simulink model "leader_qball2"  (Simulink 8.3)
settings: Solver=ode1  StartTime=0.0  StopTime=inf  FixedStep=0.002  RelTol=1e-3
InitFcn:
  | QBall_2_Setup
values from neighbouring files (symbols this model uses):
  g = 9.81    [QBall_2_System_Parameters.m]
  joystick_range_max = 0.8    [QBall_2_Setup.m]
  joystick_range_min = 0.5    [QBall_2_Setup.m]
  KdHEIGHT_DOWN = 0.15    [QBall_2_Controller_Design.m]
  KdHEIGHT_UP = 0.15    [QBall_2_Controller_Design.m]
  KdOUTER_PITCH_DOWN = 0.4    [QBall_2_Controller_Design.m]
  KdOUTER_PITCH_UP = 0.6    [QBall_2_Controller_Design.m]
  KdOUTER_ROLL_DOWN = 0.4    [QBall_2_Controller_Design.m]
  KdOUTER_ROLL_UP = 0.4    [QBall_2_Controller_Design.m]
  KdPITCH_DOWN = 0.1    [QBall_2_Controller_Design.m]
  KdPITCH_UP = 0.1    [QBall_2_Controller_Design.m]
  KdROLL_DOWN = 0.1    [QBall_2_Controller_Design.m]
  KdROLL_UP = 0.1    [QBall_2_Controller_Design.m]
  KdYAW_DOWN = 0.32    [QBall_2_Controller_Design.m]
  KdYAW_UP = 0.32    [QBall_2_Controller_Design.m]
  KiHEIGHT_DOWN = 0.35    [QBall_2_Controller_Design.m]
  KiHEIGHT_UP = 0.35    [QBall_2_Controller_Design.m]
  KiOUTER_PITCH_DOWN = 0.08    [QBall_2_Controller_Design.m]
  KiOUTER_PITCH_UP = 0.08    [QBall_2_Controller_Design.m]
  KiOUTER_ROLL_DOWN = 0.08    [QBall_2_Controller_Design.m]
  KiOUTER_ROLL_UP = 0.08    [QBall_2_Controller_Design.m]
  KiPITCH_DOWN = 0.08    [QBall_2_Controller_Design.m]
  KiPITCH_UP = 0.08    [QBall_2_Controller_Design.m]
  KiROLL_DOWN = 0.08    [QBall_2_Controller_Design.m]
  KiROLL_UP = 0.08    [QBall_2_Controller_Design.m]
  KiYAW_DOWN = 0.0    (= 0)    [QBall_2_Controller_Design.m]
  KiYAW_UP = 0.0    (= 0)    [QBall_2_Controller_Design.m]
  KpHEIGHT_DOWN = 0.5    [QBall_2_Controller_Design.m]
  KpHEIGHT_UP = 0.5    [QBall_2_Controller_Design.m]
  KpOUTER_PITCH_DOWN = 0.3    [QBall_2_Controller_Design.m]
  KpOUTER_PITCH_UP = 0.3    [QBall_2_Controller_Design.m]
  KpOUTER_ROLL_DOWN = 0.3    [QBall_2_Controller_Design.m]
  KpOUTER_ROLL_UP = 0.3    [QBall_2_Controller_Design.m]
  KpPITCH_DOWN = 0.5    [QBall_2_Controller_Design.m]
  KpPITCH_UP = 0.5    [QBall_2_Controller_Design.m]
  KpROLL_DOWN = 0.5    [QBall_2_Controller_Design.m]
  KpROLL_UP = 0.5    [QBall_2_Controller_Design.m]
  KpYAW_DOWN = 0.45    [QBall_2_Controller_Design.m]
  KpYAW_UP = 0.45    [QBall_2_Controller_Design.m]
  LIMIT_CMD_PITCH = 5*pi/180    (= 0.0872664625997)    [QBall_2_Controller_Design.m]
  LIMIT_CMD_ROLL = 5*pi/180    (= 0.0872664625997)    [QBall_2_Controller_Design.m]
  LIMIT_MAX_HEIGHT = 2    [QBall_2_Controller_Design.m]
  LIMIT_MAX_X = 1    [QBall_2_Controller_Design.m]
  LIMIT_MAX_Z = 1    [QBall_2_Controller_Design.m]
  LIMIT_MIN_HEIGHT = 0.3    [QBall_2_Controller_Design.m]
  LIMIT_MIN_X = -1    [QBall_2_Controller_Design.m]
  LIMIT_MIN_Z = -1    [QBall_2_Controller_Design.m]
  LIMIT_RATE_HEIGHT = 0.05    [QBall_2_Controller_Design.m]
  LIMIT_RATE_X = 0.15    [QBall_2_Controller_Design.m]
  LIMIT_RATE_YAW = 15*pi/180    (= 0.261799387799)    [QBall_2_Controller_Design.m]
  LIMIT_RATE_Z = 0.15    [QBall_2_Controller_Design.m]
  LIMIT_uCMD_PITCH = 0.5    [QBall_2_Controller_Design.m]
  LIMIT_uCMD_ROLL = 0.5    [QBall_2_Controller_Design.m]
  LIMIT_uCMD_YAW = 0.5    [QBall_2_Controller_Design.m]
  OFFSET_HEIGHT = 0.3    [QBall_2_System_Parameters.m]
  OMEGA_FILTER = 60    [QBall_2_System_Parameters.m]
  TRIM_THROTTLE = M*g/(4*K)    [QBall_2_Controller_Design.m]
  TRIM_U_PITCH = 0.009    [QBall_2_Controller_Design.m]
  TRIM_U_ROLL = -0.0065    [QBall_2_Controller_Design.m]
undefined symbols (not defined in the file or in its folder): DiscIntNeverNeededParam, qc_get_step_size
libraries: quarc_library x27, simulink x23
(part 1 of 3)
settings Model: Creator=jdaly  LastModifiedBy=user  SimulationMode=external  ExtModeTrigDuration=5000
settings SolverCC: PositivePriorityOrder=on
settings OptimizationCC: ExpressionDepthLimit=2147483647
settings DebuggingCC: FcnCallInpInsideContextMsg=EnableAllAsWarning
settings RTWCC: SystemTargetFile=quarc_linux_duovero.tlc  TemplateMakefile=quarc_linux_duovero_tmf  Description=QUARC Linux DuoVero Target  ProcessScript=quarc_linux_duovero_make_rtw_hook
settings STFCustomTargetCC: TargetLibSuffix=.a  TargetPreCompLibLocation=C:\PROGRA~3\QUARC\lib\2014a\LINUX_~3\release  CodeReplacementLibrary=C89/C90 (ANSI)  ConcurrentExecutionCompliant=on  GeneratePreprocessorConditionals=Disable all  CombineOutputUpdateFcns=on  CPPClassGenCompliant=on  GRTInterface=off  SystemTargetFile=quarc_linux_duovero.tlc
settings GRTTargetCC: TargetLibSuffix=.a  TargetPreCompLibLocation=C:\PROGRA~3\QUARC\lib\2014a\LINUX_~3\release  CodeReplacementLibrary=C89/C90 (ANSI)  ParMdlRefBuildCompliant=off  CompOptLevelCompliant=off  CombineOutputUpdateFcns=on  MatFileLogging=off  GRTInterface=off  ExtMode=on  ExtModeMexFile=quarc_comm  ExtModeMexArgs='-w -d /tmp -uri %u', 'tcpip://192.168.2.26:17001?keep_alive=1'

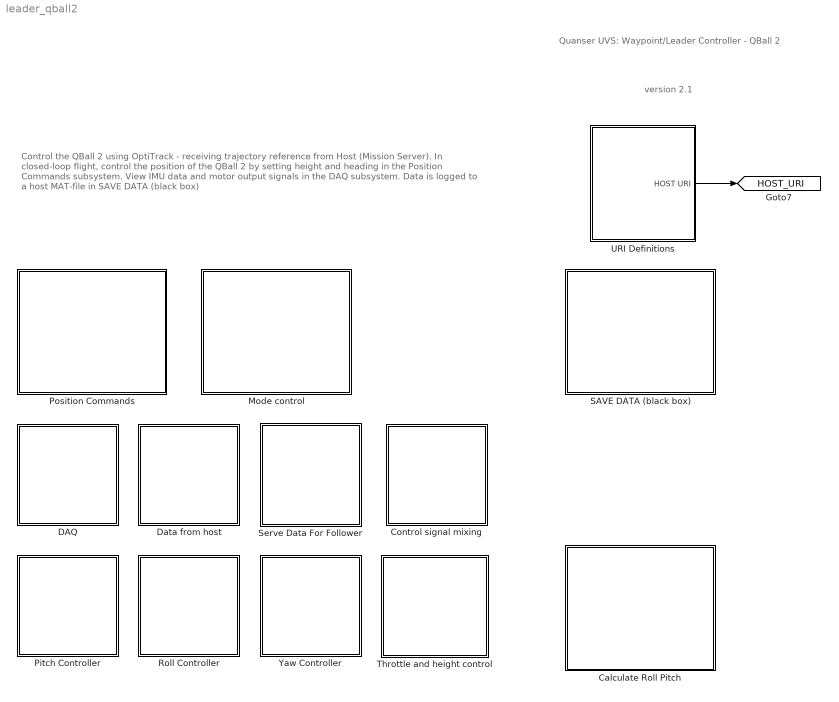
== system leader_qball2 ==
  note: Quanser UVS: Waypoint/Leader Controller - QBall 2
  note: Control the QBall 2 using OptiTrack - receiving trajectory reference
      | from Host (Mission Server).
      |
      | In closed-loop flight, control the position of the QBall 2 by setting height
      | and heading in the Position Commands subsystem.
      |
      | View IMU data and motor output signals in the DAQ subsystem.
      | Data is logged to a host MAT-file in SAVE DATA (black box)
  note: version 2.1
  Calculate Roll Pitch : Subsystem
  Control signal mixing : Subsystem
  DAQ : Subsystem
  Data from host : Subsystem
  Mode control : Subsystem
  Pitch Controller : Subsystem
  Position Commands : Subsystem
  Roll Controller : Subsystem
  SAVE DATA (black box) : Subsystem
  Serve Data For Follower : Subsystem
  Throttle and height control : Subsystem
  URI Definitions : Subsystem
  Yaw Controller : Subsystem
  tag scope: HOST_URI=global
  wires:
  URI Definitions/1(HOST URI) -> [HOST_URI]

== system leader_qball2/Calculate Roll Pitch ==
  note: Note: These calculations are obsolete (as of version 2.1). Roll and Pitch are calculated in the DAQ subsystem.
  Calculate Pitch : Subsystem
  Calculate Roll : Subsystem

== system leader_qball2/Control signal mixing ==
  note: u4 - Right
  note: u3 - Left
  note: u2 - Front
  note: u1 - Back
  Gain2 : Gain  Gain=-1
  Mux : Mux
  Safety - Motor Shutoff if: - Roll/Pitch Data Runaway (> 40 deg) - Initial 3 second of execution for motor initialization : Subsystem
  Sum : Sum  Inputs=+++
  Sum1 : Sum  Inputs=++-
  Sum2 : Sum  Inputs=+++
  Sum3 : Sum  Inputs=++-
  tag scope: motor_outputs=global
  wires:
  Sum1/1 -> Mux/2
  Sum2/1 -> Mux/3
  Sum3/1 -> Mux/4
  Mux/1 -> Safety - Motor Shutoff if: - Roll/Pitch Data Runaway (> 40 deg) - Initial 3 second of execution for motor initialization/1(motors in)
  Sum/1 -> Mux/1
  [u_pitch] -> Sum/3, Sum1/3
  [u_roll] -> Sum2/3, Sum3/3
  [u_yaw] -> Gain2/1, Sum1/2, Sum/2
  Safety - Motor Shutoff if: - Roll/Pitch Data Runaway (> 40 deg) - Initial 3 second of execution for motor initialization/1(motors) -> [motor_outputs]
  Gain2/1 -> Sum2/2, Sum3/2
  [throttle_cmd] -> Sum2/1, Sum3/1, Sum1/1, Sum/1

== system leader_qball2/DAQ ==
  note: Motor outputs: back, front, left, right
  Battery : Scope
      settings: TimeRange=5  YMin=9.9  YMax=13  SaveName=ScopeData14
  Battery (V) : Display
  HIL Initialize : quarc_library/Data Acquisition/Generic/Configuration/HIL Initialize  Priority=-99  object_name=QBall 2  board_type=qball2  board_number=0  board_options=gyro_fs=500;gyro_rate=800;gyro_bw=110;accel_rate=800;accel_fs=8  exclusive=off  active=off  hardware_clocks=[]  clock_modes=[]  initial_clock_frequencies=[]  set_clock_params_at_start=off  set_clock_params_at_switch_in=off  set_clock_frequencies_at_start=off  set_clock_frequencies_at_switch_in=off  analog_input_channels=[0:2]  analog_input_maximums=[5 5 15]  analog_input_minimums=[0 0 0]  set_analog_input_params_at_start=off  set_analog_input_params_at_switch_in=off  analog_output_channels=[]  analog_output_maximums=[]  analog_output_minimums=[]  initial_analog_outputs=[]  final_analog_outputs=[]  watchdog_analog_outputs=[]  set_analog_output_params_at_start=off  set_analog_output_params_at_switch_in=off  set_analog_outputs_at_start=off  set_analog_outputs_at_switch_in=off  set_analog_outputs_at_terminate=off  set_analog_outputs_at_switch_out=off  set_analog_outputs_on_watchdog=off  digital_input_channels=[]  digital_output_channels=[8:9]  digital_output_configuration=[]  initial_digital_outputs=[0]  final_digital_outputs=[1 1]  watchdog_digital_outputs=[0]  set_digital_output_params_at_start=off  set_digital_output_params_at_switch_in=off  set_digital_outputs_at_start=on  set_digital_outputs_at_switch_in=off  set_digital_outputs_at_terminate=on  set_digital_outputs_at_switch_out=off  set_digital_outputs_on_watchdog=on  encoder_channels=[]  quadrature=[]  encoder_filter_frequency=[]  initial_encoder_counts=[]  set_encoder_params_at_start=off  set_encoder_params_at_switch_in=off  set_encoder_counts_at_start=off  set_encoder_counts_at_switch_in=off  pwm_channels=[]  pwm_modes=[0]  pwm_frequency=20e6/1024  pwm_configuration=[0]  pwm_alignment=[0]  pwm_polarity=[1]  pwm_leading_deadband=[0]  pwm_trailing_deadband=[0]  initial_pwm_outputs=[0]  final_pwm_outputs=[0]  watchdog_pwm_outputs=[0]  set_pwm_params_at_start=on  set_pwm_params_at_switch_in=off  set_pwm_outputs_at_start=on  set_pwm_outputs_at_switch_in=off  set_pwm_outputs_at_terminate=on  set_pwm_outputs_at_switch_out=off  set_pwm_outputs_on_watchdog=on  other_output_channels=[11000:11003]  initial_other_outputs=[0]  final_other_outputs=[0]  watchdog_other_outputs=[0]  set_other_outputs_at_start=on  set_other_outputs_at_switch_in=off  set_other_outputs_at_terminate=on  set_other_outputs_at_switch_out=off  set_other_outputs_on_watchdog=on
  HIL Read Write1 : quarc_library/Data Acquisition/Generic/Immediate I//O/HIL Read Write  object_name=QBall 2  analog_output_channels=[]  pwm_output_channels=[]  digital_output_channels=[8, 9]  other_output_channels=[11003 11002 11000:11001]  analog_input_channels=[2]  encoder_input_channels=[]  digital_input_channels=[]  other_input_channels=[3000:3002 4000:4002 0]  sample_time=qc_get_step_size  active=off  vector_output=on  vector_input=on  data_type_mode=Inherit via back propagation  encoder_data_type=double  digital_data_type=boolean
      settings: AttributesFormatString=(%<object_name>)
  HIL Watchdog : quarc_library/Data Acquisition/Generic/Watchdog/HIL Watchdog  object_name=QBall 2  timeout=0.1  sample_time=qc_get_step_size  active=off
      settings: AttributesFormatString=(%<object_name>)
  Initialize sensors : Subsystem
  Low battery check : Subsystem
  Memory : Memory  X0=[0 0 0 0]
  Motor enable : Constant  Value=[1 1]
  PWM : Scope
      settings: TimeRange=5  YMin=0.46  YMax=0.68  SaveName=ScopeData8
  Sample Time : quarc_library/Sources/Time/Sample Time  Priority=-99  sample_time=qc_get_step_size
  Saturation : Saturate  UpperLimit=1  LowerLimit=0
  Select sonar : Selector  InputPortWidth=7  Indices=7
  sonar : Scope
      settings: TimeRange=5  YMin=0.8  YMax=1.4  SaveName=ScopeData34
  spike detection : Subsystem
  watchdog : Scope
      settings: TimeRange=5  YMin=0  YMax=6.5  SaveName=ScopeData32
  tag scope: pwm_output=global, sample_time=global
  wires:
  [motor_outputs] -> Memory/1
  Memory/1 -> Saturation/1
  Saturation/1 -> PWM/1, [pwm_output], HIL Read Write1/2
  Low battery check/1(v) -> Battery (V)/1, Battery/1
  Motor enable/1 -> HIL Read Write1/1
  HIL Read Write1/1 -> Low battery check/1(In1)
  HIL Watchdog/1 -> watchdog/1
  Sample Time/1 -> [sample_time]
  HIL Read Write1/2 -> Select sonar/1, Initialize sensors/1(In1)
  Select sonar/1 -> sonar/1, spike detection/1(In1)

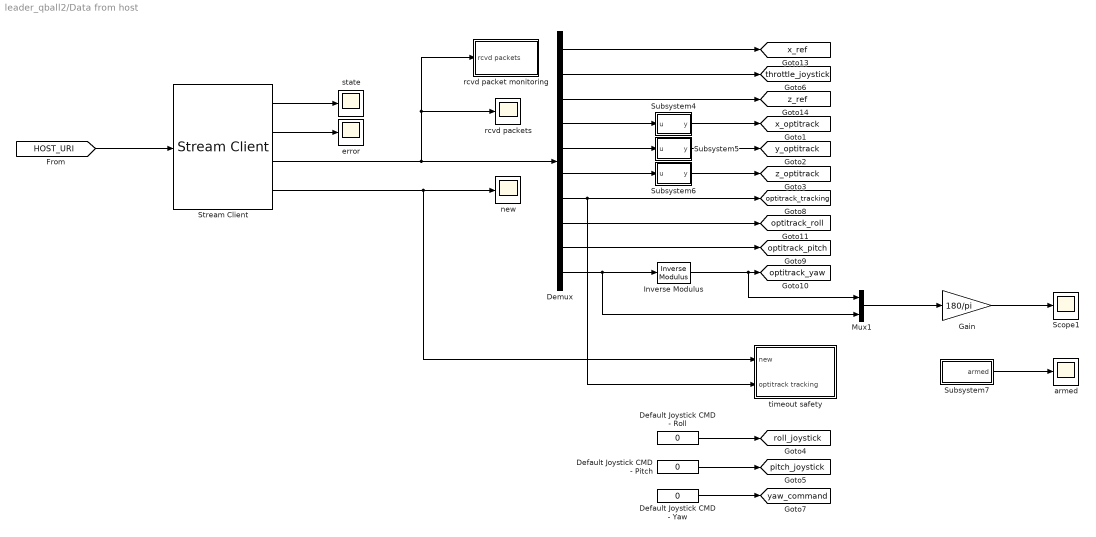
== system leader_qball2/Data from host ==
  Default Joystick CMD - Pitch : Constant  Value=0
  Default Joystick CMD - Roll : Constant  Value=0
  Default Joystick CMD - Yaw : Constant  Value=0
  Demux : Demux  Outputs=10
  Gain : Gain  Gain=180/pi
  Inverse Modulus : quarc_library/Discontinuities/Inverse Modulus  modulus=2*pi  output_derivative=off  output_revolutions=off  max_x=Inf  min_x=-Inf
  Mux1 : Mux  Inputs=2
  Scope1 : Scope
      settings: YMin=-0.48  YMax=-0.405  SaveName=InvModData1
  Stream Client : quarc_library/Communications/Basic/Stream Client  uri_source=External input port  uri=tcpip://192.168.2.15:18005  apply_uri_to_all_configs=on  send_buffer_size=1460  receive_buffer_size=1460  byte_order=little endian (Intel - LSB first)  optimization=Minimum latency  implementation=Use non-blocking I/O  send_options=Do not send data  receive_options=Receive most recent data  send_fifo_size=1000  receive_fifo_size=1000  send_priority=0  receive_priority=0  default_value=zeros(10,1)  send_dimensions=off  receive_dimensions=off  max_dimensions=-1  sample_time=qc_get_step_size  active=off  data_type=Inherited via back propagation  type_expr=BusObject
  Subsystem4 : Subsystem
  Subsystem5 : Subsystem
  Subsystem6 : Subsystem
  Subsystem7 : Subsystem
  armed : Scope
      settings: SaveName=ScopeData7
  error : Scope
      settings: TimeRange=10  YMin=-1  YMax=1  SaveName=ScopeData45
  new : Scope
      settings: SaveName=ScopeData10
  rcvd packet monitoring : Subsystem
  rcvd packets : Scope
      settings: YMin=-1  YMax=1  SaveName=ScopeData5
  state : Scope
      settings: TimeRange=10  YMin=1.9  YMax=2.1  SaveName=ScopeData13
  timeout safety : Subsystem
  tag scope: optitrack_pitch=global, optitrack_roll=global, optitrack_tracking=global, optitrack_yaw=global, pitch_joystick=global, roll_joystick=global, throttle_joystick=global, x_optitrack=global, x_ref=global, y_optitrack=global, yaw_command=global, z_optitrack=global, z_ref=global
  wires:
  Stream Client/1 -> state/1
  Stream Client/2 -> error/1
  Subsystem4/1(y) -> [x_optitrack]
  Subsystem5/1(y) -> [y_optitrack]
  Subsystem6/1(y) -> [z_optitrack]
  Stream Client/3 -> rcvd packets/1, rcvd packet monitoring/1(rcvd packets), Demux/1
  Stream Client/4 -> timeout safety/1(new), new/1
  Subsystem7/1(armed) -> armed/1
  Inverse Modulus/1 -> Mux1/1, [optitrack_yaw]
  Demux/10 -> Mux1/2, Inverse Modulus/1
  Mux1/1 -> Gain/1
  Gain/1 -> Scope1/1
  [HOST_URI] -> Stream Client/1
  Default Joystick CMD - Roll/1 -> [roll_joystick]
  Default Joystick CMD - Pitch/1 -> [pitch_joystick]
  Default Joystick CMD - Yaw/1 -> [yaw_command]
  Demux/9 -> [optitrack_pitch]
  Demux/3 -> [z_ref]
  Demux/2 -> [throttle_joystick]
  Demux/1 -> [x_ref]
  Demux/6 -> Subsystem6/1(u)
  Demux/5 -> Subsystem5/1(u)
  Demux/4 -> Subsystem4/1(u)
  Demux/8 -> [optitrack_roll]
  Demux/7 -> timeout safety/2(optitrack tracking), [optitrack_tracking]

== system leader_qball2/Mode control ==
  note: Note: the height is set to closed-loop mode using the sonar sensor.
      | You can override the height mode and use manual throttle control
      | at your own risk.
  note: Set to 0 for joystick roll and pitch control.
      | Set to 1 for autonomous position control using OptiTrack.
  note: Set to 1 for autonomous heading control using magnetometer.
      | Set to 0 for joystick yaw control.
      | NOTE: first make sure the magnetometer is calibrated and the offset is set in the field
      | HiQ\Calculate Roll Pitch Heading Height\Calculate Heading\camera frame heading offset
  CLOSED-LOOP ON : Constant
  JOYSTICK ON : Constant  Value=0
  Manual Switch2 : ManualSwitch
  Manual Switch4 : ManualSwitch
  tag scope: heading_mode=global, height_mode=global, position_mode=global
  wires:
  CLOSED-LOOP ON/1 -> Manual Switch4/1, Manual Switch2/1, [height_mode]
  JOYSTICK ON/1 -> Manual Switch4/2, Manual Switch2/2
  Manual Switch4/1 -> [heading_mode]
  Manual Switch2/1 -> [position_mode]

== system leader_qball2/Pitch Controller ==
  Gain : Gain  Gain=0.15
  Gain1 : Gain  Gain=180/pi
  Manual Switch : ManualSwitch
  Mux : Mux  Inputs=3
  Mux1 : Mux  Inputs=3
  Pitch : Scope
      settings: YMin=-0.8  YMax=1  SaveName=ScopeData3
  Pitch1 : Scope
      settings: TimeRange=40  YMin=-70  YMax=100  SaveName=ScopeData41
  Subsystem : Subsystem
  pitch controller : Subsystem
  tag scope: pitch_cmd=global
  wires:
  Subsystem/1(pitch command) -> Mux/1, Manual Switch/1
  pitch controller/1(Pitch) -> Mux/2
  Mux/1 -> Pitch/1
  [optitrack_pitch] -> Mux/3
  [pitch_Kalman] -> Mux1/1
  [pitch_comp] -> Mux1/2
  Mux1/1 -> Gain1/1
  Gain1/1 -> Pitch1/1
  [optitrack_pitch] -> Mux1/3
  [pitch_joystick] -> Gain/1
  Manual Switch/1 -> pitch controller/1(cmd), [pitch_cmd]
  Gain/1 -> Manual Switch/2

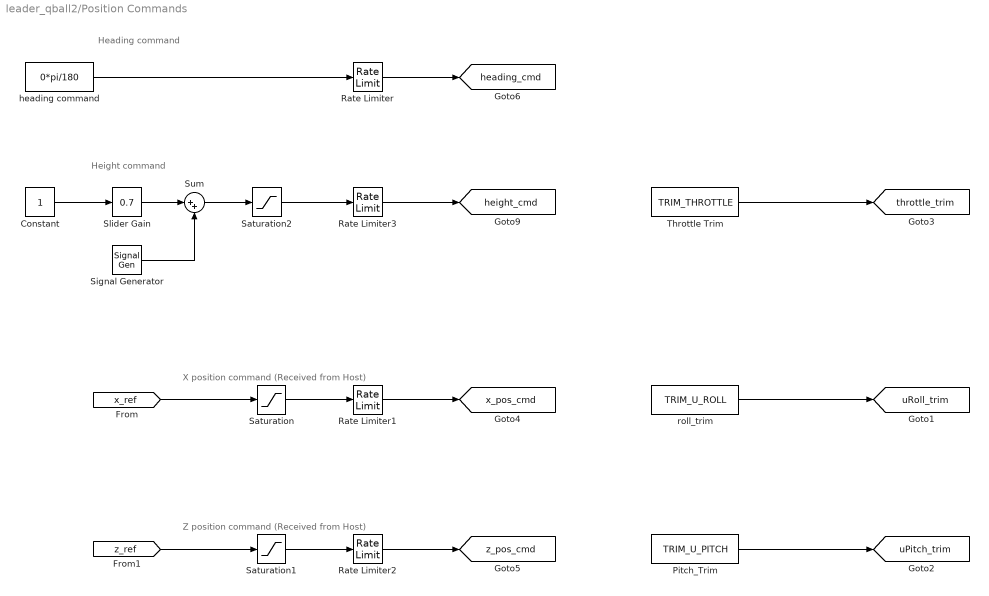
== system leader_qball2/Position Commands ==
  note: Heading command
  note: Height command
  note: X position command (Received from Host)
  note: Z position command (Received from Host)
  Constant : Constant
  Pitch_Trim : Constant  Value=TRIM_U_PITCH
  Rate Limiter : RateLimiter  RisingSlewLimit=LIMIT_RATE_YAW  FallingSlewLimit=-LIMIT_RATE_YAW  SampleTimeMode=inherited
  Rate Limiter1 : RateLimiter  RisingSlewLimit=LIMIT_RATE_X  FallingSlewLimit=-LIMIT_RATE_X  SampleTimeMode=inherited
  Rate Limiter2 : RateLimiter  RisingSlewLimit=LIMIT_RATE_Z  FallingSlewLimit=-LIMIT_RATE_Z  SampleTimeMode=inherited
  Rate Limiter3 : RateLimiter  RisingSlewLimit=LIMIT_RATE_HEIGHT  FallingSlewLimit=-LIMIT_RATE_HEIGHT  SampleTimeMode=inherited
  Saturation : Saturate  UpperLimit=LIMIT_MAX_X  LowerLimit=LIMIT_MIN_X
  Saturation1 : Saturate  UpperLimit=LIMIT_MAX_Z  LowerLimit=LIMIT_MIN_Z
  Saturation2 : Saturate  UpperLimit=LIMIT_MAX_HEIGHT  LowerLimit=LIMIT_MIN_HEIGHT
  Signal Generator : SignalGenerator  WaveForm=square  Amplitude=0  Frequency=0.0125
  Slider Gain : simulink/Math Operations/Slider Gain  low=0  gain=0.7  high=1
  Sum : Sum  Inputs=|++
  Throttle Trim : Constant  Value=TRIM_THROTTLE
  heading command : Constant  Value=0*pi/180
  roll_trim : Constant  Value=TRIM_U_ROLL
  tag scope: heading_cmd=global, height_cmd=global, throttle_trim=global, uPitch_trim=global, uRoll_trim=global, x_pos_cmd=global, z_pos_cmd=global
  wires:
  Saturation/1 -> Rate Limiter1/1
  Saturation1/1 -> Rate Limiter2/1
  Constant/1 -> Slider Gain/1
  heading command/1 -> Rate Limiter/1
  Slider Gain/1 -> Sum/1
  Sum/1 -> Saturation2/1
  Signal Generator/1 -> Sum/2
  Rate Limiter/1 -> [heading_cmd]
  Saturation2/1 -> Rate Limiter3/1
  Rate Limiter1/1 -> [x_pos_cmd]
  Rate Limiter2/1 -> [z_pos_cmd]
  Rate Limiter3/1 -> [height_cmd]
  Throttle Trim/1 -> [throttle_trim]
  roll_trim/1 -> [uRoll_trim]
  Pitch_Trim/1 -> [uPitch_trim]
  [x_ref] -> Saturation/1
  [z_ref] -> Saturation1/1

== system leader_qball2/Roll Controller ==
  Gain : Gain  Gain=0.15
  Gain1 : Gain  Gain=180/pi
  Gain4 : Gain  Gain=180/pi
  Manual Switch : ManualSwitch
  Mux : Mux
  Mux1 : Mux
  Roll : Scope
      settings: TimeRange=40  YMin=0  YMax=47.5  SaveName=ScopeData9
  Roll Controller : Subsystem
  Roll1 : Scope
      settings: TimeRange=40  YMin=-60  YMax=100  SaveName=ScopeData40
  Subsystem : Subsystem
  tag scope: roll_cmd=global
  wires:
  Subsystem/1(roll command) -> Mux/1, Manual Switch/1
  Mux/1 -> Gain4/1
  Roll Controller/1(Roll) -> Mux/2
  [optitrack_roll] -> Mux/3
  [roll_Kalman] -> Mux/4
  Gain4/1 -> Roll/1
  [roll_Kalman] -> Mux1/1
  [roll_comp] -> Mux1/2
  Mux1/1 -> Gain1/1
  Gain1/1 -> Roll1/1
  [optitrack_roll] -> Mux1/3
  [roll_acc] -> Mux1/4
  Manual Switch/1 -> [roll_cmd], Roll Controller/1(cmd)
  [roll_joystick] -> Gain/1
  Gain/1 -> Manual Switch/2

== system leader_qball2/SAVE DATA (black box) ==
  note: Saves the data to a MAT file on the host PC. Note that the model must be connected
      | in external mode and stopped correctly for the MAT file to be saved.
      | Append signals to the end of the mux block to save additional signals.
      | Each time the model is run it saves a new file with the data and time appended
      | to the file name.
      |
      | Signals can be read after stopping the model by first loading the MAT file, then plotting
      | the data signals. NOTE: data points are saved in rows, with the first row always containing
      | the time signal - so add 1 to the index of the signals listed here. E.g.,
      |
      | load qball_flight_data.mat
      | t = qball_data(1,:);
      | roll = qball_data(22,:);
      | plot(t, roll);
  Mux1 : Mux  Inputs=7
  Signals 1-10 : Subsystem
  Signals 11-20 : Subsystem
  Signals 21-30 : Subsystem
  Signals 31-40 : Subsystem
  Signals 41-50 : Subsystem
  Signals 51-60 : Subsystem
  Signals 61-70 : Subsystem
  To Host File : quarc_library/Sinks/To Host/To Host File  file_name=qball_flight_data_%{date}_%{time}.mat  variable_name=qball_data  decimation=1  sample_time=-1  file_format=MAT-file v.4  options=No header or footer  append=off  final_file_name=qball_flight_data_20-Aug-2015_16-55-50.mat
      settings: AttributesFormatString=%<file_name>
  wires:
  Mux1/1 -> To Host File/1
  Signals 41-50/1(Out1) -> Mux1/5
  Signals 31-40/1(Out1) -> Mux1/4
  Signals 21-30/1(Out1) -> Mux1/3
  Signals 11-20/1(Out1) -> Mux1/2
  Signals 1-10/1(Out1) -> Mux1/1
  Signals 51-60/1(Out1) -> Mux1/6
  Signals 61-70/1(Out1) -> Mux1/7

== system leader_qball2/Serve Data For Follower ==
  Display1 : Display
      settings: Decimation=100
  Display2 : Display
      settings: Decimation=100
  Display3 : Display
      settings: Decimation=100
  Dummy Heading Reference (rad) : Constant  Value=0
  Enable : Constant
  Mux : Mux  Inputs=3
  Stream Server : quarc_library/Communications/Basic/Stream Server  uri_source=Specify via dialog (do not evaluate)  uri=tcpip://localhost:18007  apply_uri_to_all_configs=on  send_buffer_size=1460  receive_buffer_size=1460  byte_order=little endian (Intel - LSB first)  optimization=Minimum latency  implementation=Use non-blocking I/O  send_options=Send most recent data  receive_options=Do not receive data  send_fifo_size=1000  receive_fifo_size=1000  send_priority=0  receive_priority=0  default_value=[0]  send_dimensions=off  receive_dimensions=off  max_dimensions=-1  sample_time=qc_get_step_size  active=off  data_type=Inherited via back propagation  type_expr=BusObject
      settings: AttributesFormatString="\"tcpip://localhost:18007\""
  wires:
  Mux/1 -> Stream Server/1
  Enable/1 -> Stream Server/2
  Stream Server/3 -> Display3/1
  Stream Server/2 -> Display2/1
  Stream Server/1 -> Display1/1
  [z_optitrack] -> Mux/2
  [x_optitrack] -> Mux/1
  Dummy Heading Reference (rad)/1 -> Mux/3

== system leader_qball2/Throttle and height control ==
  Height joystick adjust : Subsystem
  Joystick mode throttle : Subsystem
  "Safety - Active During Emergency Landing: Ramp Throttle CMD down to zero if Sonar Failed " : Subsystem
  Switch : Switch  Threshold=0.5
  height control : Subsystem
  throttle cmd : Scope
      settings: YMin=0  YMax=1.1  SaveName=ScopeData19
  throttle sw : Scope
      settings: YMin=0.05  YMax=0.1  SaveName=ScopeData27
  tag scope: throttle_cmd=global
  wires:
  Height joystick adjust/1(cmd out) -> height control/1(height command)
  Switch/1 -> throttle sw/1, "Safety - Active During Emergency Landing: Ramp Throttle CMD down to zero if Sonar Failed "/1(throttle)
  height control/1(throttle) -> Switch/1
  Joystick mode throttle/1(throttle) -> Switch/3
  [height_mode] -> Switch/2
  "Safety - Active During Emergency Landing: Ramp Throttle CMD down to zero if Sonar Failed "/1(Out1) -> throttle cmd/1, [throttle_cmd]
  [height_cmd] -> Height joystick adjust/1(cmd)

== system leader_qball2/URI Definitions ==
  note: Note: Make sure QBall 2 IP address match the intended active unit in the following places:
      | - Under Simulation->Model Configuration Parameters->Code Generation->Interface->MEX-file arguments
  note: Default URI:
      |
      | HOST Server to LEADER: tcpip://192.168.2.222:18006
      | HOST Server to FOLLOWER: tcpip://192.168.2.222:18005
      | LEADER Server to FOLLOWER: tcpip://192.168.30:18007
      |
      | Leader/Waypoint Control Model URI:
      | tcpip://192.168.2.22:17001?nagle=no,keep_alive=1
  note: Define Communications URI Here
  String Constant1 : quarc_library/Strings/String Constant  string_value=tcpip://192.168.2.10:18006  evaluate_string=off  string_type=text  max_length=80  sample_time=inf  variable_size=off
      settings: AttributesFormatString="\"tcpip://192.168.2.10:18006\""
  HOST URI : Outport
  wires:
  String Constant1/1 -> HOST URI/1

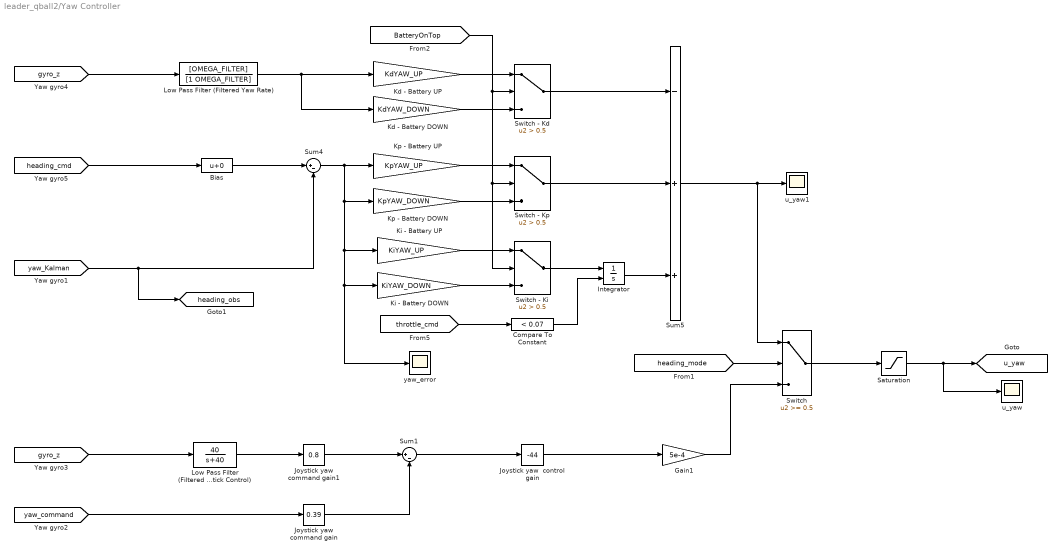
== system leader_qball2/Yaw Controller ==
  Bias : Bias
  Compare To Constant : simulink/Logic and Bit Operations/Compare To Constant  relop=<  const=0.07  OutDataTypeStr=boolean  ZeroCross=off
  Gain1 : Gain  Gain=5e-4
  Integrator : Integrator  ExternalReset=level
  Joystick yaw  control gain : simulink/Math Operations/Slider Gain  low=-100  gain=-44  high=0
  Joystick yaw command gain : simulink/Math Operations/Slider Gain  low=0  gain=0.39  high=0.6
  Joystick yaw command gain1 : simulink/Math Operations/Slider Gain  low=-1  gain=0.8  high=1
  Kd - Battery DOWN : Gain  Gain=KdYAW_DOWN
  Kd - Battery UP : Gain  Gain=KdYAW_UP
  Ki - Battery DOWN : Gain  Gain=KiYAW_DOWN
  Ki - Battery UP : Gain  Gain=KiYAW_UP
  Kp - Battery DOWN : Gain  Gain=KpYAW_DOWN
  Kp - Battery UP : Gain  Gain=KpYAW_UP
  Low Pass Filter (Filtered Yaw Rate) : TransferFcn  Numerator=[OMEGA_FILTER]  Denominator=[1 OMEGA_FILTER]
  Low Pass Filter (Filtered Yaw Rate) (For Joytstick Control) : TransferFcn  Numerator=[40]  Denominator=[1 40]
  Saturation : Saturate  UpperLimit=LIMIT_uCMD_YAW  LowerLimit=-LIMIT_uCMD_YAW
  Sum1 : Sum  Inputs=|+-
  Sum4 : Sum  Inputs=|+-
  Sum5 : Sum  Inputs=-++
  Switch : Switch  Threshold=0.5
  Switch - Kd : Switch  Criteria=u2 > Threshold  Threshold=0.5
  Switch - Ki : Switch  Criteria=u2 > Threshold  Threshold=0.5
  Switch - Kp : Switch  Criteria=u2 > Threshold  Threshold=0.5
  u_yaw : Scope
      settings: YMin=-0.0225  YMax=0.02  SaveName=ScopeData4
  u_yaw1 : Scope
      settings: YMin=2.93e-05  YMax=3.15e-05  SaveName=ScopeData23
  yaw_error : Scope
      settings: YMin=-0.1005  YMax=-0.091  SaveName=ScopeData24
  tag scope: heading_obs=global, u_yaw=global
  wires:
  [yaw_command] -> Joystick yaw command gain/1
  Sum1/1 -> Joystick yaw  control gain/1
  [heading_mode] -> Switch/2
  Switch/1 -> Saturation/1
  Joystick yaw command gain/1 -> Sum1/2
  Joystick yaw  control gain/1 -> Gain1/1
  Gain1/1 -> Switch/3
  Sum4/1 -> Kp - Battery DOWN/1, Ki - Battery UP/1, Ki - Battery DOWN/1, yaw_error/1, Kp - Battery UP/1
  Sum5/1 -> Switch/1, u_yaw1/1
  [yaw_Kalman] -> Sum4/2, [heading_obs]
  Saturation/1 -> [u_yaw], u_yaw/1
  [gyro_z] -> Low Pass Filter (Filtered Yaw Rate) (For Joytstick Control)/1
  Low Pass Filter (Filtered Yaw Rate) (For Joytstick Control)/1 -> Joystick yaw command gain1/1
  Joystick yaw command gain1/1 -> Sum1/1
  [heading_cmd] -> Bias/1
  Compare To Constant/1 -> Integrator/2
  [throttle_cmd] -> Compare To Constant/1
  [gyro_z] -> Low Pass Filter (Filtered Yaw Rate)/1
  Low Pass Filter (Filtered Yaw Rate)/1 -> Kd - Battery UP/1, Kd - Battery DOWN/1
  Integrator/1 -> Sum5/3
  Bias/1 -> Sum4/1
  Kd - Battery UP/1 -> Switch - Kd/1
  Kd - Battery DOWN/1 -> Switch - Kd/3
  [BatteryOnTop] -> Switch - Kp/2, Switch - Ki/2, Switch - Kd/2
  Kp - Battery UP/1 -> Switch - Kp/1
  Kp - Battery DOWN/1 -> Switch - Kp/3
  Switch - Kd/1 -> Sum5/1
  Switch - Kp/1 -> Sum5/2
  Ki - Battery UP/1 -> Switch - Ki/1
  Ki - Battery DOWN/1 -> Switch - Ki/3
  Switch - Ki/1 -> Integrator/1

== system leader_qball2/Calculate Roll Pitch/Calculate Pitch ==
  Fcn : Fcn  Expr=asin(u/9.81)
  HPF : TransferFcn  Numerator=[2 0]  Denominator=[2 1]
  Integrator : Integrator
  LPF : TransferFcn  Numerator=1  Denominator=[2 1]
  Sum2 : Sum
  Terminator : Terminator
  tag scope: pitch=global, pitch_comp=global
  wires:
  [accel_x] -> Fcn/1
  Integrator/1 -> HPF/1
  HPF/1 -> Sum2/2, [pitch_comp]
  LPF/1 -> Sum2/1
  Fcn/1 -> [pitch], LPF/1
  [gyro_y] -> Integrator/1
  Sum2/1 -> Terminator/1

== system leader_qball2/Calculate Roll Pitch/Calculate Roll ==
  Fcn : Fcn  Expr=asin(u/9.81)
  Gain1 : Gain  Gain=-1
  HPF1 : TransferFcn  Numerator=[2 0]  Denominator=[2 1]
  Integrator : Integrator
  LPF1 : TransferFcn  Numerator=1  Denominator=[2 1]
  Manual Switch : ManualSwitch
  Sum3 : Sum
  Switch : Switch  Threshold=0.5
  Terminator : Terminator
  tag scope: roll=global, roll_comp=global
  wires:
  [accel_y] -> Gain1/1
  Gain1/1 -> Fcn/1
  [gyro_x] -> Integrator/1
  Integrator/1 -> HPF1/1
  Fcn/1 -> LPF1/1, [roll]
  LPF1/1 -> Sum3/1
  HPF1/1 -> Sum3/2, Manual Switch/1
  [optitrack_tracking] -> Switch/2
  Sum3/1 -> Switch/3
  [optitrack_roll] -> Switch/1
  Switch/1 -> Terminator/1
  Manual Switch/1 -> [roll_comp]
  [roll_acc] -> Manual Switch/2

== system leader_qball2/Control signal mixing/Safety - Motor Shutoff if: - Roll/Pitch Data Runaway (> 40 deg) - Initial 3 second of execution for motor initialization ==
  note: Check that pitch and roll are always less than 40 degrees.
      | If pitch or roll exceeds 40 degrees it is a runaway condition
      | and the motors should be stopped.
  motors in : Inport
  Abs : Abs
  Abs1 : Abs
  Compare To Constant1 : simulink/Logic and Bit Operations/Compare To Constant  relop=>  const=40*pi/180  OutDataTypeStr=uint8  ZeroCross=off
  Compare To Constant2 : simulink/Logic and Bit Operations/Compare To Constant  relop=>  const=40*pi/180  OutDataTypeStr=uint8  ZeroCross=off
  Enabled Subsystem : Subsystem  TreatAsAtomicUnit=on
  Logical Operator : Logic  Operator=OR  AllPortsSameDT=off  OutDataTypeStr=boolean
  Product1 : Product  Inputs=3  OutDataTypeStr=double  RndMeth=Zero
  Product2 : Product  OutDataTypeStr=double  RndMeth=Zero
  "Roll, Pitch runaway check" : Scope
      settings: SaveName=ScopeData38
  Step Initialize zero throttle for 3 seconds : Step  Time=3  SampleTime=0
  motors_in : Scope
      settings: SaveName=ScopeData50
  motors_out : Scope
      settings: SaveName=ScopeData51
  throttle enable : Subsystem
  motors : Outport
  wires:
  motors in/1 -> motors_in/1, Product1/2
  throttle enable/1(en) -> Product1/1
  [roll_comp] -> Abs1/1
  [pitch_comp] -> Abs/1
  Compare To Constant1/1 -> Logical Operator/1
  Compare To Constant2/1 -> Logical Operator/2
  Logical Operator/1 -> Enabled Subsystem/Enable
  Enabled Subsystem/1(Out1) -> "Roll, Pitch runaway check"/1, Product1/3
  Product1/1 -> Product2/2
  Abs/1 -> Compare To Constant1/1
  Abs1/1 -> Compare To Constant2/1
  Step Initialize zero throttle for 3 seconds/1 -> Product2/1
  Product2/1 -> motors_out/1, motors/1

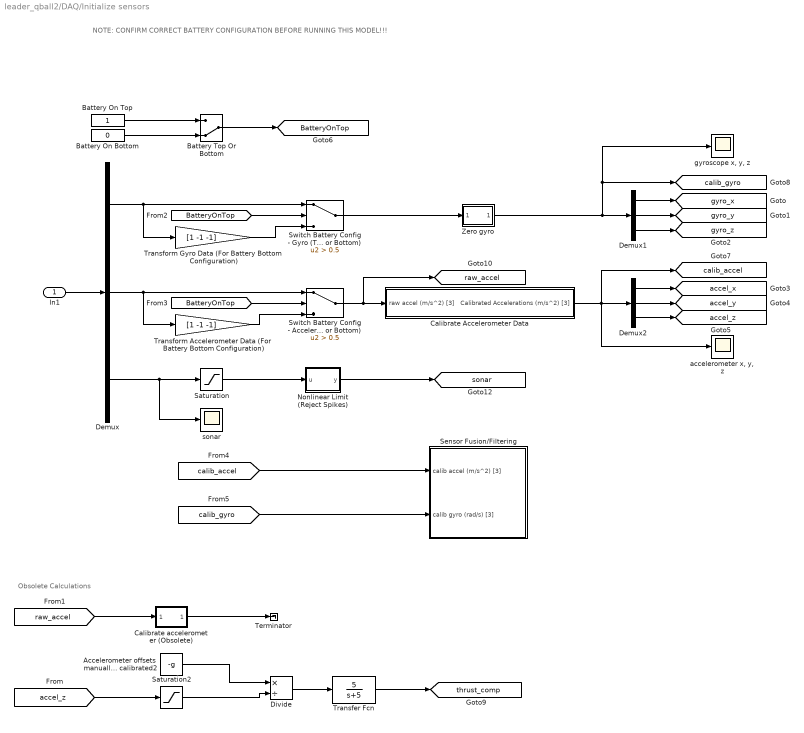
== system leader_qball2/DAQ/Initialize sensors ==
  note: Obsolete Calculations
  note: NOTE: CONFIRM CORRECT BATTERY
      | CONFIGURATION BEFORE RUNNING
      | THIS MODEL!!!
  In1 : Inport
  Accelerometer offsets manually calibrated2 : Constant  Value=-g
  Battery On Bottom : Constant  Value=0
  Battery On Top : Constant
  Battery Top Or Bottom : ManualSwitch  CurrentSetting=0
  Calibrate Accelerometer Data : Subsystem
  Calibrate accelerometer (Obsolete) : Subsystem
  Demux : Demux  Outputs=[3 3 1]
  Demux1 : Demux  Outputs=3
  Demux2 : Demux  Outputs=3
  Divide : Product  Inputs=*/
  Nonlinear Limit (Reject Spikes) : Subsystem
  Saturation : Saturate  UpperLimit=3  LowerLimit=0
  Saturation2 : Saturate  UpperLimit=-9.0  LowerLimit=-9.8
  Sensor Fusion/Filtering : Subsystem
  Switch Battery Config - Acceleromter (Top or Bottom) : Switch  Criteria=u2 > Threshold  Threshold=0.5
  Switch Battery Config - Gyro (Top or Bottom) : Switch  Criteria=u2 > Threshold  Threshold=0.5
  Terminator : Terminator
  Transfer Fcn : TransferFcn  Numerator=[5]  Denominator=[1 5]
  Transform Accelerometer Data (For Battery Bottom Configuration) : Gain  Gain=[1 -1 -1]
  Transform Gyro Data (For Battery Bottom Configuration) : Gain  Gain=[1 -1 -1]
  Zero gyro : Subsystem
  "accelerometer x, y, z" : Scope
      settings: TimeRange=5  YMin=-10  YMax=3  SaveName=ScopeData31
  "gyroscope x, y, z" : Scope
      settings: TimeRange=5  YMin=-0.125  YMax=0.425  SaveName=ScopeData30
  sonar : Scope
      settings: YMin=0.1  YMax=1.9  SaveName=ScopeData15
  tag scope: BatteryOnTop=global, accel_x=global, accel_y=global, accel_z=global, calib_accel=global, calib_gyro=global, gyro_x=global, gyro_y=global, gyro_z=global, raw_accel=global, sonar=global, thrust_comp=global
  wires:
  Demux1/1 -> [gyro_x]
  Demux1/2 -> [gyro_y]
  Demux1/3 -> [gyro_z]
  Demux2/1 -> [accel_x]
  Demux2/2 -> [accel_y]
  Demux2/3 -> [accel_z]
  Accelerometer offsets manually calibrated2/1 -> Divide/1
  Divide/1 -> Transfer Fcn/1
  Transfer Fcn/1 -> [thrust_comp]
  In1/1 -> Demux/1
  Saturation/1 -> Nonlinear Limit (Reject Spikes)/1(u)
  Nonlinear Limit (Reject Spikes)/1(y) -> [sonar]
  Saturation2/1 -> Divide/2
  [accel_z] -> Saturation2/1
  [raw_accel] -> Calibrate accelerometer (Obsolete)/1(In1)
  Calibrate accelerometer (Obsolete)/1(Out1) -> Terminator/1
  Demux/3 -> sonar/1, Saturation/1
  [BatteryOnTop] -> Switch Battery Config - Gyro (Top or Bottom)/2
  Transform Gyro Data (For Battery Bottom Configuration)/1 -> Switch Battery Config - Gyro (Top or Bottom)/3
  Demux/2 -> Switch Battery Config - Acceleromter (Top or Bottom)/1, Transform Accelerometer Data (For Battery Bottom Configuration)/1
  [BatteryOnTop] -> Switch Battery Config - Acceleromter (Top or Bottom)/2
  Transform Accelerometer Data (For Battery Bottom Configuration)/1 -> Switch Battery Config - Acceleromter (Top or Bottom)/3
  Switch Battery Config - Gyro (Top or Bottom)/1 -> Zero gyro/1(In1)
  [calib_gyro] -> Sensor Fusion/Filtering/2(calib gyro (rad/s) [3])
  [calib_accel] -> Sensor Fusion/Filtering/1(calib accel (m/s^2) [3])
  Switch Battery Config - Acceleromter (Top or Bottom)/1 -> [raw_accel], Calibrate Accelerometer Data/1(raw accel (m/s^2) [3])
  Demux/1 -> Transform Gyro Data (For Battery Bottom Configuration)/1, Switch Battery Config - Gyro (Top or Bottom)/1
  Zero gyro/1(Out1) -> Demux1/1, "gyroscope x, y, z"/1, [calib_gyro]
  Calibrate Accelerometer Data/1(Calibrated Accelerations (m/s^2) [3]) -> "accelerometer x, y, z"/1, Demux2/1, [calib_accel]
  Battery On Bottom/1 -> Battery Top Or Bottom/2
  Battery On Top/1 -> Battery Top Or Bottom/1
  Battery Top Or Bottom/1 -> [BatteryOnTop]

== system leader_qball2/DAQ/Low battery check ==
  In1 : Inport
  Compare To Constant : simulink/Logic and Bit Operations/Compare To Constant  relop=<=  const=10.5  OutDataTypeStr=uint8  ZeroCross=off
  Show Message on Host : quarc_library/Sinks/Error Handling/Show Message on Host  message_type=Fixed error message  message_icon=Warning  message=Low battery!
      settings: AttributesFormatString="\"%<message>\""
  v : Outport
  tag scope: battery_voltage=global
  wires:
  In1/1 -> [battery_voltage], v/1, Compare To Constant/1
  Compare To Constant/1 -> Show Message on Host/1

== system leader_qball2/DAQ/spike detection ==
  In1 : Inport
  Abs : Abs
  Compare To Constant : simulink/Logic and Bit Operations/Compare To Constant  relop=>=  const=3  OutDataTypeStr=boolean  ZeroCross=off
  Show Message on Host1 : quarc_library/Sinks/Error Handling/Show Message on Host  message_type=Fixed error message  message_icon=Warning  message=Spike detected on Sonar data!
      settings: AttributesFormatString="\"%<message>\""
  wires:
  Abs/1 -> Compare To Constant/1
  Compare To Constant/1 -> Show Message on Host1/1
  In1/1 -> Abs/1

== system leader_qball2/Data from host/Subsystem4 ==
  u : Inport
  Constant : Constant  Value=3
  Embedded MATLAB Function : MATLAB Function  TreatAsAtomicUnit=on
  Memory : Memory
  y : Outport
  wires:
  Embedded MATLAB Function/1(y) -> Memory/1, y/1
  Memory/1 -> Embedded MATLAB Function/2(x)
  u/1 -> Embedded MATLAB Function/1(u)
  Constant/1 -> Embedded MATLAB Function/3(threshold)

== system leader_qball2/Data from host/Subsystem5 ==
  u : Inport
  Constant : Constant  Value=3
  Embedded MATLAB Function : MATLAB Function  TreatAsAtomicUnit=on
  Memory : Memory
  y : Outport
  wires:
  Constant/1 -> Embedded MATLAB Function/3(threshold)
  u/1 -> Embedded MATLAB Function/1(u)
  Memory/1 -> Embedded MATLAB Function/2(x)
  Embedded MATLAB Function/1(y) -> y/1, Memory/1

== system leader_qball2/Data from host/Subsystem6 ==
  u : Inport
  Constant : Constant  Value=3
  Embedded MATLAB Function : MATLAB Function  TreatAsAtomicUnit=on
  Memory : Memory
  y : Outport
  wires:
  Embedded MATLAB Function/1(y) -> Memory/1, y/1
  Memory/1 -> Embedded MATLAB Function/2(x)
  u/1 -> Embedded MATLAB Function/1(u)
  Constant/1 -> Embedded MATLAB Function/3(threshold)

== system leader_qball2/Data from host/Subsystem7 ==
  Clock : Clock
  Compare To Constant : simulink/Logic and Bit Operations/Compare To Constant  relop=>  const=5  OutDataTypeStr=boolean  ZeroCross=off
  Compare To Constant1 : simulink/Logic and Bit Operations/Compare To Constant  relop=>  const=0.1  OutDataTypeStr=boolean  ZeroCross=off
  Logical Operator : Logic  AllPortsSameDT=off  OutDataTypeStr=boolean
  armed : Outport
  tag scope: armed=global
  wires:
  Clock/1 -> Compare To Constant/1
  [throttle_joystick] -> Compare To Constant1/1
  Compare To Constant/1 -> Logical Operator/1
  Compare To Constant1/1 -> Logical Operator/2
  Logical Operator/1 -> armed/1, [armed]

== system leader_qball2/Data from host/rcvd packet monitoring ==
  rcvd packets : Inport
  Packet from Target : Scope
      settings: TimeRange=10  YMin=-0.05  YMax=1  SaveName=ScopeData18
  spike detection : Subsystem
  wires:
  rcvd packets/1 -> Packet from Target/1, spike detection/1(In1)

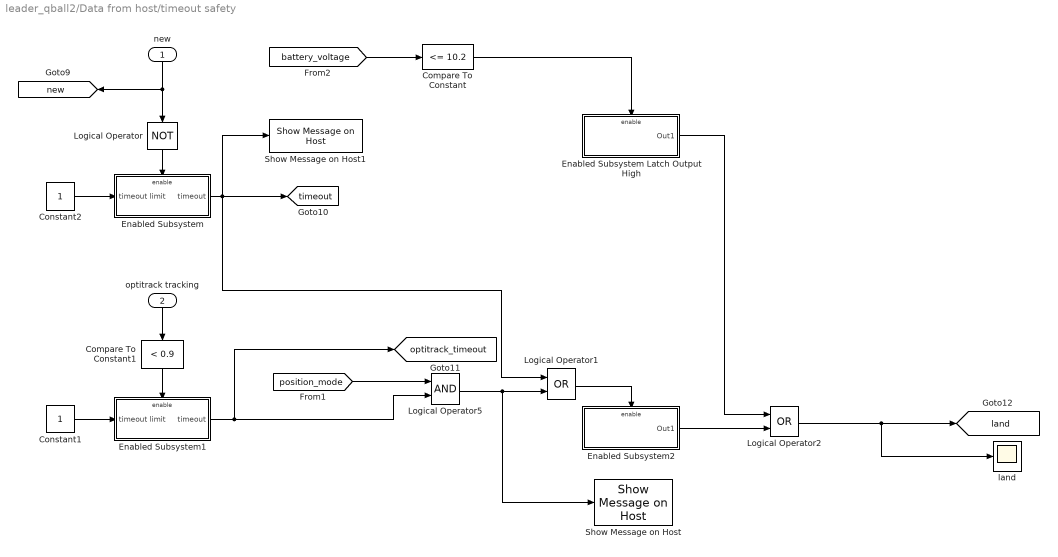
== system leader_qball2/Data from host/timeout safety ==
  new : Inport
  optitrack tracking : Inport  Port=2
  Compare To Constant : simulink/Logic and Bit Operations/Compare To Constant  relop=<=  const=10.2  OutDataTypeStr=uint8
  Compare To Constant1 : simulink/Logic and Bit Operations/Compare To Constant  relop=<  const=0.9  OutDataTypeStr=boolean
  Constant1 : Constant
  Constant2 : Constant
  Enabled Subsystem : Subsystem  TreatAsAtomicUnit=on
  Enabled Subsystem1 : Subsystem  TreatAsAtomicUnit=on
  Enabled Subsystem2 : Subsystem  TreatAsAtomicUnit=on
  Enabled Subsystem Latch Output High : Subsystem  TreatAsAtomicUnit=on
  Logical Operator : Logic  Operator=NOT  AllPortsSameDT=off  OutDataTypeStr=boolean
  Logical Operator1 : Logic  Operator=OR  AllPortsSameDT=off  OutDataTypeStr=boolean
  Logical Operator2 : Logic  Operator=OR  AllPortsSameDT=off  OutDataTypeStr=boolean
  Logical Operator5 : Logic  AllPortsSameDT=off  OutDataTypeStr=boolean
  Show Message on Host : quarc_library/Sinks/Error Handling/Show Message on Host  message_type=Fixed error message  message_icon=Warning  message=OptiTrack is not tracking the marker!
      settings: AttributesFormatString="\"%<message>\""
  Show Message on Host1 : quarc_library/Sinks/Error Handling/Show Message on Host  message_type=Fixed error message  message_icon=Warning  message=Host connection timeout detected!
      settings: AttributesFormatString="\"%<message>\""
  land : Scope
      settings: SaveName=ScopeData6
  tag scope: land=global, new=global, optitrack_timeout=global, timeout=global
  wires:
  Logical Operator1/1 -> Enabled Subsystem2/Enable
  Logical Operator5/1 -> Show Message on Host/1, Logical Operator1/2
  [position_mode] -> Logical Operator5/1
  optitrack tracking/1 -> Compare To Constant1/1
  Constant1/1 -> Enabled Subsystem1/1(timeout limit)
  Enabled Subsystem1/1(timeout) -> [optitrack_timeout], Logical Operator5/2
  Compare To Constant1/1 -> Enabled Subsystem1/Enable
  new/1 -> Logical Operator/1, [new]
  Constant2/1 -> Enabled Subsystem/1(timeout limit)
  Enabled Subsystem/1(timeout) -> Show Message on Host1/1, Logical Operator1/1, [timeout]
  Logical Operator/1 -> Enabled Subsystem/Enable
  Enabled Subsystem2/1(Out1) -> Logical Operator2/2
  [battery_voltage] -> Compare To Constant/1
  Logical Operator2/1 -> [land], land/1
  Compare To Constant/1 -> Enabled Subsystem Latch Output High/Enable
  Enabled Subsystem Latch Output High/1(Out1) -> Logical Operator2/1

== system leader_qball2/Pitch Controller/Subsystem ==
  Joystick Sensitivity : Gain  Gain=0.15
  OT pos control : Subsystem
  Safety - Emergency Landing Zero Ref CMD : Subsystem
  Switch : Switch  Threshold=0.5
  pitch command : Outport
  wires:
  [pitch_joystick] -> Joystick Sensitivity/1
  Switch/1 -> Safety - Emergency Landing Zero Ref CMD/1(In1)
  OT pos control/1(pitch cmd) -> Switch/1
  Joystick Sensitivity/1 -> Switch/3
  [position_mode] -> Switch/2
  Safety - Emergency Landing Zero Ref CMD/1(Out1) -> pitch command/1

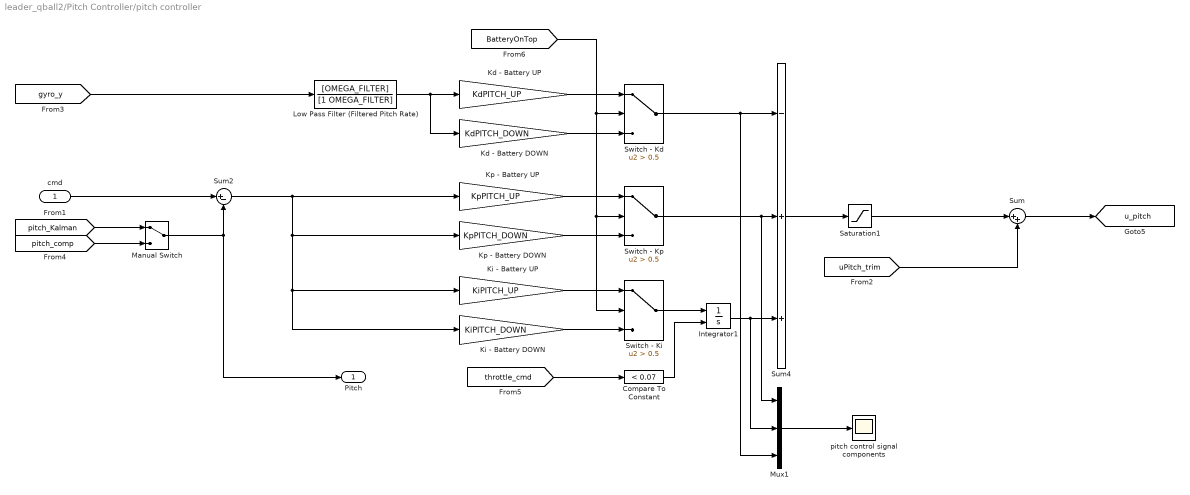
== system leader_qball2/Pitch Controller/pitch controller ==
  cmd : Inport
  Compare To Constant : simulink/Logic and Bit Operations/Compare To Constant  relop=<  const=0.07  OutDataTypeStr=boolean  ZeroCross=off
  Integrator1 : Integrator  ExternalReset=level
  Kd - Battery DOWN : Gain  Gain=KdPITCH_DOWN
  Kd - Battery UP : Gain  Gain=KdPITCH_UP
  Ki - Battery DOWN : Gain  Gain=KiPITCH_DOWN
  Ki - Battery UP : Gain  Gain=KiPITCH_UP
  Kp - Battery DOWN : Gain  Gain=KpPITCH_DOWN
  Kp - Battery UP : Gain  Gain=KpPITCH_UP
  Low Pass Filter (Filtered Pitch Rate) : TransferFcn  Numerator=[OMEGA_FILTER]  Denominator=[1 OMEGA_FILTER]
  Manual Switch : ManualSwitch
  Mux1 : Mux  Inputs=3
  Saturation1 : Saturate  UpperLimit=LIMIT_uCMD_PITCH  LowerLimit=-LIMIT_uCMD_PITCH
  Sum : Sum  Inputs=|++
  Sum2 : Sum  Inputs=|+-
  Sum4 : Sum  Inputs=-++
  Switch - Kd : Switch  Criteria=u2 > Threshold  Threshold=0.5
  Switch - Ki : Switch  Criteria=u2 > Threshold  Threshold=0.5
  Switch - Kp : Switch  Criteria=u2 > Threshold  Threshold=0.5
  pitch control signal components : Scope
      settings: SaveName=ScopeData2
  Pitch : Outport
  tag scope: u_pitch=global
  wires:
  Compare To Constant/1 -> Integrator1/2
  [throttle_cmd] -> Compare To Constant/1
  [gyro_y] -> Low Pass Filter (Filtered Pitch Rate)/1
  [pitch_comp] -> Manual Switch/2
  [pitch_Kalman] -> Manual Switch/1
  Saturation1/1 -> Sum/1
  Sum/1 -> [u_pitch]
  [uPitch_trim] -> Sum/2
  Low Pass Filter (Filtered Pitch Rate)/1 -> Kd - Battery UP/1, Kd - Battery DOWN/1
  Integrator1/1 -> Mux1/2, Sum4/3
  cmd/1 -> Sum2/1
  Sum2/1 -> Kp - Battery UP/1, Kp - Battery DOWN/1, Ki - Battery UP/1, Ki - Battery DOWN/1
  Manual Switch/1 -> Pitch/1, Sum2/2
  Sum4/1 -> Saturation1/1
  Mux1/1 -> pitch control signal components/1
  Kd - Battery UP/1 -> Switch - Kd/1
  Kd - Battery DOWN/1 -> Switch - Kd/3
  [BatteryOnTop] -> Switch - Kd/2, Switch - Kp/2, Switch - Ki/2
  Switch - Kd/1 -> Mux1/3, Sum4/1
  Switch - Kp/1 -> Mux1/1, Sum4/2
  Kp - Battery DOWN/1 -> Switch - Kp/3
  Kp - Battery UP/1 -> Switch - Kp/1
  Ki - Battery DOWN/1 -> Switch - Ki/3
  Ki - Battery UP/1 -> Switch - Ki/1
  Switch - Ki/1 -> Integrator1/1

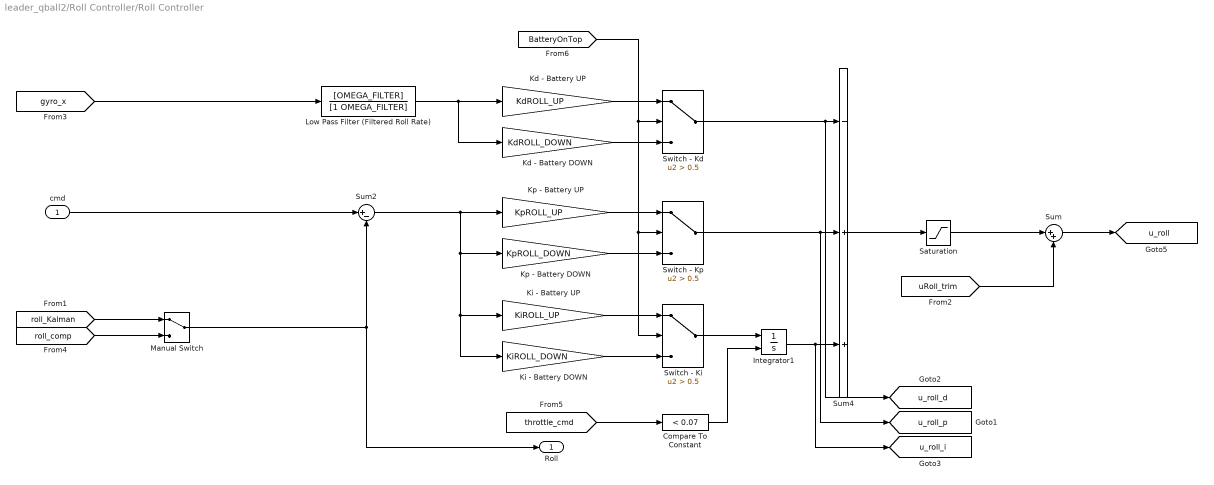
== system leader_qball2/Roll Controller/Roll Controller ==
  cmd : Inport
  Compare To Constant : simulink/Logic and Bit Operations/Compare To Constant  relop=<  const=0.07  OutDataTypeStr=boolean  ZeroCross=off
  Integrator1 : Integrator  ExternalReset=level
  Kd - Battery DOWN : Gain  Gain=KdROLL_DOWN
  Kd - Battery UP : Gain  Gain=KdROLL_UP
  Ki - Battery DOWN : Gain  Gain=KiROLL_DOWN
  Ki - Battery UP : Gain  Gain=KiROLL_UP
  Kp - Battery DOWN : Gain  Gain=KpROLL_DOWN
  Kp - Battery UP : Gain  Gain=KpROLL_UP
  Low Pass Filter (Filtered Roll Rate) : TransferFcn  Numerator=[OMEGA_FILTER]  Denominator=[1 OMEGA_FILTER]
  Manual Switch : ManualSwitch
  Saturation : Saturate  UpperLimit=LIMIT_uCMD_ROLL  LowerLimit=-LIMIT_uCMD_ROLL
  Sum : Sum  Inputs=|++
  Sum2 : Sum  Inputs=|+-
  Sum4 : Sum  Inputs=-++
  Switch - Kd : Switch  Criteria=u2 > Threshold  Threshold=0.5
  Switch - Ki : Switch  Criteria=u2 > Threshold  Threshold=0.5
  Switch - Kp : Switch  Criteria=u2 > Threshold  Threshold=0.5
  Roll : Outport
  tag scope: u_roll=global, u_roll_d=global, u_roll_i=global, u_roll_p=global
  wires:
  [throttle_cmd] -> Compare To Constant/1
  [gyro_x] -> Low Pass Filter (Filtered Roll Rate)/1
  [roll_Kalman] -> Manual Switch/1
  [roll_comp] -> Manual Switch/2
  Manual Switch/1 -> Sum2/2, Roll/1
  Saturation/1 -> Sum/1
  Sum/1 -> [u_roll]
  [uRoll_trim] -> Sum/2
  Compare To Constant/1 -> Integrator1/2
  Integrator1/1 -> [u_roll_i], Sum4/3
  Low Pass Filter (Filtered Roll Rate)/1 -> Kd - Battery DOWN/1, Kd - Battery UP/1
  cmd/1 -> Sum2/1
  Sum2/1 -> Kp - Battery DOWN/1, Ki - Battery UP/1, Ki - Battery DOWN/1, Kp - Battery UP/1
  Sum4/1 -> Saturation/1
  Kd - Battery UP/1 -> Switch - Kd/1
  Kd - Battery DOWN/1 -> Switch - Kd/3
  Switch - Kd/1 -> [u_roll_d], Sum4/1
  Kp - Battery UP/1 -> Switch - Kp/1
  Kp - Battery DOWN/1 -> Switch - Kp/3
  [BatteryOnTop] -> Switch - Kp/2, Switch - Ki/2, Switch - Kd/2
  Switch - Kp/1 -> [u_roll_p], Sum4/2
  Switch - Ki/1 -> Integrator1/1
  Ki - Battery DOWN/1 -> Switch - Ki/3
  Ki - Battery UP/1 -> Switch - Ki/1

== system leader_qball2/Roll Controller/Subsystem ==
  Joystick Sensitivity : Gain  Gain=0.15
  OT pos control : Subsystem
  Safety - Emergency Landing Zero Ref CMD : Subsystem
  Switch : Switch  Threshold=0.5
  roll command : Outport
  wires:
  [roll_joystick] -> Joystick Sensitivity/1
  Safety - Emergency Landing Zero Ref CMD/1(Out1) -> roll command/1
  [position_mode] -> Switch/2
  OT pos control/1(roll cmd) -> Switch/1
  Joystick Sensitivity/1 -> Switch/3
  Switch/1 -> Safety - Emergency Landing Zero Ref CMD/1(In1)

== system leader_qball2/SAVE DATA (black box)/Signals 1-10 ==
  note: 5
  note: 1-4
  note: 6
  note: 7
  note: 8
  note: 9
  note: 10
  Mux : Mux  Inputs=7
  Out1 : Outport
  wires:
  Mux/1 -> Out1/1
  [gyro_x] -> Mux/2
  [pwm_output] -> Mux/1
  [gyro_y] -> Mux/3
  [gyro_z] -> Mux/4
  [accel_x] -> Mux/5
  [accel_y] -> Mux/6
  [accel_z] -> Mux/7

== system leader_qball2/SAVE DATA (black box)/Signals 11-20 ==
  note: 20
  note: 11
  note: 12
  note: 17
  note: 18
  note: 19
  Mux : Mux  Inputs=10
  Out1 : Outport
  wires:
  [sonar] -> Mux/1
  Mux/1 -> Out1/1
  [battery_voltage] -> Mux/2
  [roll_Kalman] -> Mux/7
  [pitch_Kalman] -> Mux/8
  [roll_cmd] -> Mux/9
  [pitch_cmd] -> Mux/10
  [height_rate_estimate] -> Mux/4
  [h_cmd] -> Mux/3
  [u_height_d] -> Mux/5
  [u_height_i] -> Mux/6

== system leader_qball2/SAVE DATA (black box)/Signals 21-30 ==
  note: 30
  note: 21
  Mux1 : Mux  Inputs=10
  Out1 : Outport
  wires:
  [roll] -> Mux1/1
  [pitch] -> Mux1/2
  [heading_obs] -> Mux1/3
  [throttle_joystick] -> Mux1/5
  [x_pos_cmd] -> Mux1/6
  [z_pos_cmd] -> Mux1/7
  [height_cmd] -> Mux1/8
  [x_optitrack] -> Mux1/9
  [y_optitrack] -> Mux1/10
  Mux1/1 -> Out1/1
  [yaw_Kalman] -> Mux1/4

== system leader_qball2/SAVE DATA (black box)/Signals 31-40 ==
  note: 31
  note: 40
  Data Type Conversion{,1..3} (4 alike) : DataTypeConversion
  Mux1 : Mux  Inputs=10
  Out1 : Outport
  wires:
  [new] -> Data Type Conversion/1
  [timeout] -> Data Type Conversion1/1
  [optitrack_timeout] -> Data Type Conversion2/1
  [land] -> Data Type Conversion3/1
  [z_optitrack] -> Mux1/1
  [optitrack_tracking] -> Mux1/2
  Data Type Conversion/1 -> Mux1/3
  Data Type Conversion1/1 -> Mux1/6
  Data Type Conversion2/1 -> Mux1/7
  [sonar] -> Mux1/8
  Data Type Conversion3/1 -> Mux1/9
  [throttle_cmd] -> Mux1/10
  Mux1/1 -> Out1/1
  [height_Kalman] -> Mux1/4
  [height_above_ground] -> Mux1/5

== system leader_qball2/SAVE DATA (black box)/Signals 41-50 ==
  note: 41
  Mux1 : Mux  Inputs=10
  Out1 : Outport
  wires:
  Mux1/1 -> Out1/1
  [height_mode] -> Mux1/1
  [heading_mode] -> Mux1/2
  [position_mode] -> Mux1/3
  [u_roll] -> Mux1/4
  [u_pitch] -> Mux1/5
  [u_yaw] -> Mux1/6
  [optitrack_roll] -> Mux1/7
  [optitrack_pitch] -> Mux1/8
  [optitrack_yaw] -> Mux1/9
  [sample_time] -> Mux1/10

== system leader_qball2/SAVE DATA (black box)/Signals 51-60 ==
  note: 51
  Demux : Demux
  Mux1 : Mux  Inputs=10
  Out1 : Outport
  wires:
  [gyro_y] -> Mux1/6
  [gyro_x] -> Mux1/5
  [pitch_comp] -> Mux1/4
  [roll_comp] -> Mux1/3
  [roll_cmd_d] -> Mux1/2
  [roll_cmd_p] -> Mux1/1
  Mux1/1 -> Out1/1
  [motor_outputs] -> Demux/1
  Demux/1 -> Mux1/7
  Demux/2 -> Mux1/8
  Demux/3 -> Mux1/9
  Demux/4 -> Mux1/10

== system leader_qball2/SAVE DATA (black box)/Signals 61-70 ==
  note: 61
  Demux : Demux
  Mux1 : Mux  Inputs=10
  Out1 : Outport
  wires:
  Demux/4 -> Mux1/10
  Demux/3 -> Mux1/9
  Demux/2 -> Mux1/8
  Demux/1 -> Mux1/7
  [motor_outputs] -> Demux/1
  Mux1/1 -> Out1/1
  [u_roll_p] -> Mux1/1
  [u_roll_d] -> Mux1/2
  [u_roll_i] -> Mux1/3
  [x_ref] -> Mux1/4
  [z_ref] -> Mux1/5
  [gyro_y] -> Mux1/6

== system leader_qball2/Throttle and height control/Height joystick adjust ==
  cmd : Inport
  Constant : Constant  Value=0
  Constant1 : Constant  Value=qc_get_step_size
  MATLAB Function : MATLAB Function  TreatAsAtomicUnit=on
  Switch : Switch  Threshold=0.5
  cmd out : Outport
  wires:
  Switch/1 -> cmd out/1
  Constant/1 -> Switch/3
  cmd/1 -> Switch/1
  [throttle_joystick] -> MATLAB Function/1(throttle)
  Constant1/1 -> MATLAB Function/2(step_size)
  MATLAB Function/1(enable) -> Switch/2

== system leader_qball2/Throttle and height control/Joystick mode throttle ==
  Divide : Product  Inputs=**
  Joystick throttle scaling : Gain  Gain=0.8
  Joystick to Throttle  Mapping : MATLAB Function  TreatAsAtomicUnit=on
  height command1 : Constant  Value=joystick_range_min
  height command2 : Constant  Value=joystick_range_max
  throttle joystick : Scope
      settings: YMin=0.45  YMax=1  SaveName=ScopeData26
  throttle : Outport
  wires:
  Divide/1 -> Joystick to Throttle  Mapping/1(u)
  [throttle_joystick] -> throttle joystick/1, Divide/2
  [thrust_comp] -> Divide/1
  height command2/1 -> Joystick to Throttle  Mapping/3(l2)
  height command1/1 -> Joystick to Throttle  Mapping/2(l1)
  Joystick to Throttle  Mapping/1(y) -> Joystick throttle scaling/1
  Joystick throttle scaling/1 -> throttle/1
